simulink model "TestStructure"  (R2023b)
settings: Solver=FixedStepDiscrete  StartTime=0.0  StopTime=inf  FixedStep=SampleTime  RelTol=1e-3
InitFcn:
  | SampleTime = 0.001;
  | ButtonValue=0;
  | load("BusConfig.mat");
undefined symbols (not defined in the file): DiscIntNeverNeededParam
libraries: slrealtimeethercatlib x219, dspfdesign x28, dspstat3 x23, simulink x21, slpidlib x10, dspswit3 x8, commfilt2 x2, dspsigops x1
(part 1 of 8)
settings Model: SimulationMode=external  ExtModeEnableFloating=off  Creator=My-Dell-PC  LastModifiedBy=My-Dell-PC
settings SolverCC: ConcurrentTasks=on  PositivePriorityOrder=on
settings OptimizationCC: BlockReduction=off  OptimizeBlockIOStorage=off  ReuseModelBlockBuffer=off
settings DebuggingCC: TasksWithSamePriorityMsg=none
settings HardwareCC: ProdBitPerLong=64  ProdLongLongMode=on  ProdHWDeviceType=Intel->x86-64 (Linux 64)
settings RTWCC: Description=Simulink Real-Time  SystemTargetFile=slrealtime.tlc  TemplateMakefile=slrealtime_default_tmf  Toolchain=Simulink Real-Time Toolchain  BuildConfiguration=Faster Runs  CodeExecutionProfiling=on  TargetLang=C++
settings CodeAppCC: MaxIdLength=128

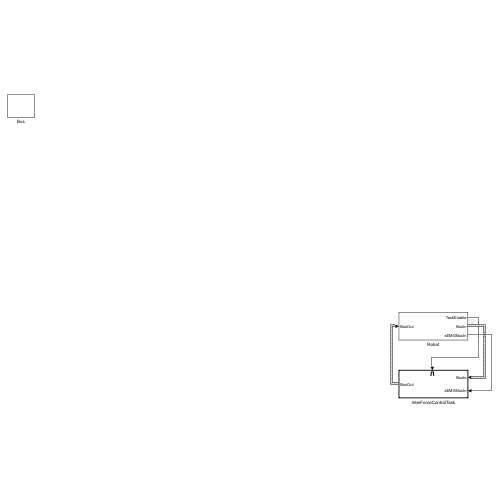
[thumbnail: Simulink's stored preview of the top-level diagram]
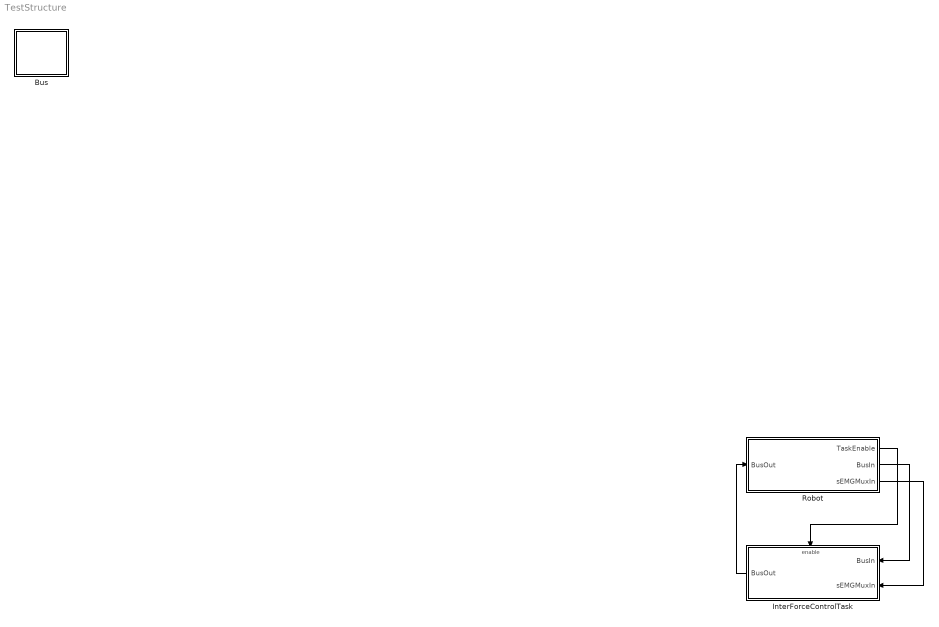
== system TestStructure ==
  Bus : Subsystem  mask{Parameter1=0}
  InterForceControlTask : Subsystem  TreatAsAtomicUnit=on
  Robot : Subsystem  InitFcn=|
      | LeftHipMotorPosDefault = -134217728;                %Unit: Cnt
      | RightHipMotorPosDefault = -134217728;               %Unit: Cnt
      | LeftHipMotor_InitPos_Degree = 185;           %Unit: Degree
      | RightHipMotor_InitPos_Degree = 58;          %Unit: Degree
      | LeftHipMotorSensorCh1FDirection = -1;       %Unit: None        1 or -1, 0 for not use
      | RightHipMotorSensorCh1FDirection = 1;      %Unit: None        1 or -1, 0 for not use
      | LeftHipMotorPosProtectUpperLim = 0;        %Unit: Degree      both Upper and lower lim config to 0 for no protect
      | LeftHipMotorPosProtectLowerLim = 0;        %Unit: Degree      both Upper and lower lim config to 0 for no protect
      | RightHipMotorPosProtectUpperLim = 0;       %Unit: Degree      both Upper and lower lim config to 0 for no protect
      | RightHipMotorPosProtectLowerLim = 0;       %Unit: Degree      both Upper and lower lim config to 0 for no protect
  wires:
  Robot/2(BusIn) -> InterForceControlTask/1(BusIn)
  Robot/1(TaskEnable) -> InterForceControlTask/Enable
  InterForceControlTask/1(BusOut) -> Robot/1(BusOut)
  Robot/3(sEMGMuxIn) -> InterForceControlTask/2(sEMGMuxIn)

== system TestStructure/Bus ==
  Subsystem : Subsystem
  Subsystem1 : Subsystem
  Subsystem4 : Subsystem
  Subsystem5 : Subsystem
  Subsystem6 : Subsystem
  Subsystem7 : Subsystem

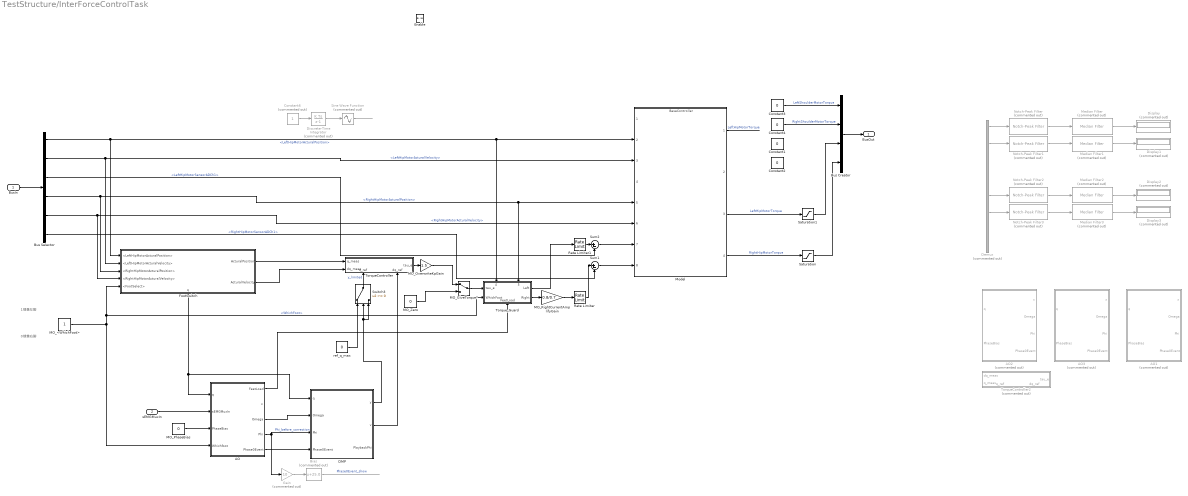
== system TestStructure/InterForceControlTask ==
  note: 0镜像右脚
  note: 1镜像左脚
  BusIn : Inport  OutDataTypeStr=Bus: SensingBusNew  BusOutputAsStruct=on
  sEMGMuxIn : Inport  Port=2
  Enable : EnablePort
  AO : Subsystem
  AO1 : Subsystem  Commented=on
  AO2 : Subsystem  Commented=on
  AO3 : Subsystem  Commented=on
  Bias : Bias  Commented=on  Bias=25.0  SaturateOnIntegerOverflow=off
  Bus Creator : BusCreator  Inputs=4  OutDataTypeStr=Bus: ControlBusNew  NonVirtualBus=on
  Bus Selector : BusSelector  OutputSignals=LeftHipMotorActuralPosition,LeftHipMotorActuralVelocity,LeftHipMotorSensorADCh1,RightHipMotorActuralPosition,RightHipMotorActuralVelocity,RightHipMotorSensorADCh1
  Constant{1..4} (4 alike) : Constant  Value=0
  Constant6 : Constant  Commented=on
  DMP : Subsystem
  Demux : Demux  Commented=on  Outputs=8
  Discrete-Time Integrator : DiscreteIntegrator  Commented=on  SampleTime=-1  ICPrevOutput=DiscIntNeverNeededParam  ICPrevScaledInput=DiscIntNeverNeededParam
  Display{,1..3} (4 alike) : Display  Commented=on
  FootSwitch : Subsystem
      settings: PortSchema="{\"entries\":[{\"content\":{\"sides\":[{\"content\":{\"connectorIds\":[\"In1\",\"In2\",\"In3\",\"In4\",\"In5\"]},\"type\":\"ConnectorPlacement.EquallySpacedRectSide\",\"uuid\":\"7ecdb0d1-44f7-4cb8-804e-f6057fee00e3\"},{\"content\":{\"connectorIds\":[\"Out1\",\"Out2\"],\"side\":\"RIGHT\"},\"type\":\"ConnectorPlacement.EquallySpacedRectSide\",\"uuid\":\"b63e60e1-496e-4124-94d3-4dbeb666215a\"},{\"content\":{\"side\":\"TOP\"},\"type\":\"ConnectorPlacement.EquallySpacedRectSide\",\"uuid\":\"11a332ee-5b07-4fe6-93fe-1398bc56bf27\"},{\"content\":{\"connectorIds\":[\"Out3\"],\"side\":\"BOTTOM\"},\"type\":\"ConnectorPlacement.EquallySpacedRectSide\",\"uuid\":\"ff7a2680-cae9-4957-8a73-46cd45583629\"}]},\"type\":\"ConnectorPlacement.EquallySpacedConnector\",\"uuid\":\"1c496143-d045-4bb8-a283-2b92538bf384\"}],\"packageUris\":[\"http://schema.mathworks.com/mf0/Connector/R2020b\"],\"version\":\"1.0\"}"
  Gain : Gain  Commented=on  Gain=10
  MO_<WhichFoot> : Constant
  MO_GiveTorque? : ManualSwitch
  MO_OverwriteKpGain : Gain  Gain=1.5
  MO_PhaseBias : Constant  Value=0
  MO_RightCurrentAmplifyGain : Gain  Gain=0.8/0.7
  MO_Zero : Constant  Value=0
  Median Filter{,1..3} (4 alike) : dspstat3/Median Filter  Commented=on  WindowLength=5  SimulateUsing=Interpreted execution
      settings: LibrarySourceBlock=|
      | dspfdesign/Median
      | Filter
  Model : ModelReference  ModelNameDialog=BaseController.slxp  ModelReferenceVersion=3.421  CopyOfModelProtected=on
  Notch-Peak Filter{,1..3} (4 alike) : dspfdesign/Notch-Peak Filter  Commented=on  Specification=Quality factor and center frequency  BandwidthPort=on  Bandwidth=2205  QualityFactorPort=off  QualityFactor=5  CenterFrequencyPort=off  CenterFrequency=50  BandwidthCoefficientPort=off  BandwidthCoefficient=0.72654  CenterFrequencyCoefficientPort=off  CenterFrequencyCoefficient=0  Output=Notch  InheritSampleRate=off  SampleRate=1000  SimulateUsing=Code generation
  Rate Limiter : RateLimiter  RisingSlewLimit=60  FallingSlewLimit=-60  SampleTimeMode=inherited
  Rate Limiter1 : RateLimiter  RisingSlewLimit=60  FallingSlewLimit=-60  SampleTimeMode=inherited
  Saturation : Saturate  UpperLimit=20  LowerLimit=-20
  Saturation1 : Saturate  UpperLimit=20  LowerLimit=-20
  Sine Wave Function : Sin  Commented=on  TimeSource=Use external signal  Amplitude=30  Bias=-30  Frequency=2*pi*0.5  Phase=0.5*pi  SampleTime=0
  Sum1 : Sum  Inputs=|+-
  Sum2 : Sum  Inputs=|+-
  Switch3 : Switch  SaturateOnIntegerOverflow=off  InputSameDT=off
  TorqueController : Subsystem
      settings: PortSchema="{\"entries\":[{\"content\":{\"sides\":[{\"content\":{\"connectorIds\":[\"In1\",\"In2\"]},\"type\":\"ConnectorPlacement.EquallySpacedRectSide\",\"uuid\":\"a70f4d3f-71f0-4d44-86b2-84ae6c965d36\"},{\"content\":{\"connectorIds\":[\"Out1\"],\"side\":\"RIGHT\"},\"type\":\"ConnectorPlacement.EquallySpacedRectSide\",\"uuid\":\"94df1563-b6d2-45fb-b198-7d0905a4894a\"},{\"content\":{\"side\":\"TOP\"},\"type\":\"ConnectorPlacement.EquallySpacedRectSide\",\"uuid\":\"a4abfadc-4e4d-4360-b10c-eb4f639dc4a4\"},{\"content\":{\"connectorIds\":[\"In3\",\"In4\"],\"side\":\"BOTTOM\"},\"type\":\"ConnectorPlacement.EquallySpacedRectSide\",\"uuid\":\"0f098f5c-7d68-4c78-935c-71623c896b5b\"}]},\"type\":\"ConnectorPlacement.EquallySpacedConnector\",\"uuid\":\"e58753f5-b0b7-4189-98c1-665b5fbcbb59\"}],\"packageUris\":[\"http://schema.mathworks.com/mf0/Connector/R2020b\"],\"version\":\"1.0\"}"
  TorqueController2 : Subsystem  Commented=on
      settings: PortSchema="{\"entries\":[{\"content\":{\"sides\":[{\"content\":{\"connectorIds\":[\"In1\",\"In2\"]},\"type\":\"ConnectorPlacement.EquallySpacedRectSide\",\"uuid\":\"a70f4d3f-71f0-4d44-86b2-84ae6c965d36\"},{\"content\":{\"connectorIds\":[\"Out1\"],\"side\":\"RIGHT\"},\"type\":\"ConnectorPlacement.EquallySpacedRectSide\",\"uuid\":\"94df1563-b6d2-45fb-b198-7d0905a4894a\"},{\"content\":{\"side\":\"TOP\"},\"type\":\"ConnectorPlacement.EquallySpacedRectSide\",\"uuid\":\"a4abfadc-4e4d-4360-b10c-eb4f639dc4a4\"},{\"content\":{\"connectorIds\":[\"In3\",\"In4\"],\"side\":\"BOTTOM\"},\"type\":\"ConnectorPlacement.EquallySpacedRectSide\",\"uuid\":\"0f098f5c-7d68-4c78-935c-71623c896b5b\"}]},\"type\":\"ConnectorPlacement.EquallySpacedConnector\",\"uuid\":\"e58753f5-b0b7-4189-98c1-665b5fbcbb59\"}],\"packageUris\":[\"http://schema.mathworks.com/mf0/Connector/R2020b\"],\"version\":\"1.0\"}"
  Torque_Guard : Subsystem
      settings: PortSchema="{\"entries\":[{\"content\":{\"sides\":[{\"content\":{\"connectorIds\":[\"In1\"]},\"type\":\"ConnectorPlacement.EquallySpacedRectSide\",\"uuid\":\"1d23c2d1-211b-4c47-b88b-c8f5a33413bd\"},{\"content\":{\"connectorIds\":[\"In4\",\"In5\"],\"side\":\"RIGHT\"},\"type\":\"ConnectorPlacement.EquallySpacedRectSide\",\"uuid\":\"4048f38c-2874-4094-b8f6-a75ec179b5c6\"},{\"content\":{\"connectorIds\":[\"In2\",\"In3\"],\"side\":\"TOP\"},\"type\":\"ConnectorPlacement.EquallySpacedRectSide\",\"uuid\":\"5dc62aa6-b4b6-4778-a65d-61d1e67b5e0a\"},{\"content\":{\"connectorIds\":[\"Out1\",\"Out2\"],\"side\":\"BOTTOM\"},\"type\":\"ConnectorPlacement.EquallySpacedRectSide\",\"uuid\":\"4577c0a2-eb02-4748-b343-e51a2d06d9c8\"}]},\"type\":\"ConnectorPlacement.EquallySpacedConnector\",\"uuid\":\"b262622a-1d3e-4ad6-baa7-9b3b8428161e\"}],\"packageUris\":[\"http://schema.mathworks.com/mf0/Connector/R2020b\"],\"version\":\"1.0\"}"
  ref_q_max : Constant  Value=0
  BusOut : Outport  OutDataTypeStr=Bus: ControlBusNew  BusOutputAsStruct=on
  wires:
  Bus Creator/1 -> BusOut/1
  Model/1 -> ?  "LeftHipMotorTorque"
  BusIn/1 -> Bus Selector/1
  Constant3/1 -> Bus Creator/1  "LeftShoulderMotorTorque"
  Model/4 -> Saturation/1  "RightHipMotorTorque"
  Constant4/1 -> Bus Creator/2  "RightShoulderMotorTorque"
  Sum2/1 -> Model/7
  Bus Selector/4 -> FootSwitch/3(<RightHipMotorActuralPosition>), Torque_Guard/5(<RightHipMotorActuralPosition>), Model/5  "<RightHipMotorActuralPosition>"
  Bus Selector/5 -> FootSwitch/4(<RightHipMotorActuralVelocity>), Model/6  "<RightHipMotorActuralVelocity>"
  Bus Selector/2 -> FootSwitch/2(<LeftHipMotorActuralVelocity>), Model/3  "<LeftHipMotorActuralVelocity>"
  Bus Selector/3 -> Sum2/2  "<LeftHipMotorSensorADCh1>"
  Bus Selector/6 -> Sum1/2  "<RightHipMotorSensorADCh1>"
  Constant6/1 -> Discrete-Time Integrator/1
  Discrete-Time Integrator/1 -> Sine Wave Function/1
  Sine Wave Function/1 -> ?
  Median Filter3/1 -> Display3/1
  Notch-Peak Filter2/1 -> Median Filter2/1
  Demux/2 -> Notch-Peak Filter1/1
  Median Filter1/1 -> Display1/1
  Notch-Peak Filter3/1 -> Median Filter3/1
  Notch-Peak Filter/1 -> Median Filter/1
  Demux/5 -> Notch-Peak Filter2/1
  Median Filter2/1 -> Display2/1
  Demux/1 -> Notch-Peak Filter/1
  Median Filter/1 -> Display/1
  Notch-Peak Filter1/1 -> Median Filter1/1
  Demux/6 -> Notch-Peak Filter3/1
  MO_PhaseBias/1 -> AO/3(PhaseBias)
  AO/4(Phi) -> DMP/3(Phi), Gain/1  "Phi_before_correction"
  AO/5(Phase0Event) -> DMP/4(Phase0Event)
  DMP/2(v) -> TorqueController/4(dq_ref)
  AO/3(Omega) -> DMP/2(Omega)
  Bus Selector/1 -> FootSwitch/1(<LeftHipMotorActuralPosition>), Model/2, Torque_Guard/4(<LeftHipMotorActuralPosition>)  "<LeftHipMotorActuralPosition>"
  Saturation/1 -> Bus Creator/4
  Model/3 -> Saturation1/1  "LeftHipMotorTorque"
  Saturation1/1 -> Bus Creator/3
  Gain/1 -> Bias/1
  Bias/1 -> ?  "Phase0Event_show"
  MO_Zero/1 -> MO_GiveTorque?/2
  TorqueController/1(tau_e) -> MO_OverwriteKpGain/1
  Sum1/1 -> Model/8
  sEMGMuxIn/1 -> AO/2(sEMGMuxIn)
  FootSwitch/3(q) -> DMP/1(q), AO/1(q)
  FootSwitch/1(ActuralPosition) -> TorqueController/1(q_meas)
  FootSwitch/2(ActuralVelocity) -> TorqueController/2(dq_meas)
  MO_GiveTorque?/1 -> Torque_Guard/3(tau_e)
  Torque_Guard/2(Left) -> Rate Limiter1/1
  Torque_Guard/1(Right) -> MO_RightCurrentAmplifyGain/1
  MO_<WhichFoot>/1 -> FootSwitch/5(<FootSelect>), Torque_Guard/2(WhichFoot), AO/4(Whichfoot)  "<WhichFoot>"
  Rate Limiter/1 -> Sum1/1
  AO/1(FeetLoad) -> Torque_Guard/1(FeetLoad)
  DMP/1(y) -> Switch3/3, Switch3/2
  ref_q_max/1 -> Switch3/1
  Switch3/1 -> TorqueController/3(q_ref)  "y_limited"
  MO_OverwriteKpGain/1 -> MO_GiveTorque?/1
  MO_RightCurrentAmplifyGain/1 -> Rate Limiter/1
  Rate Limiter1/1 -> Sum2/1

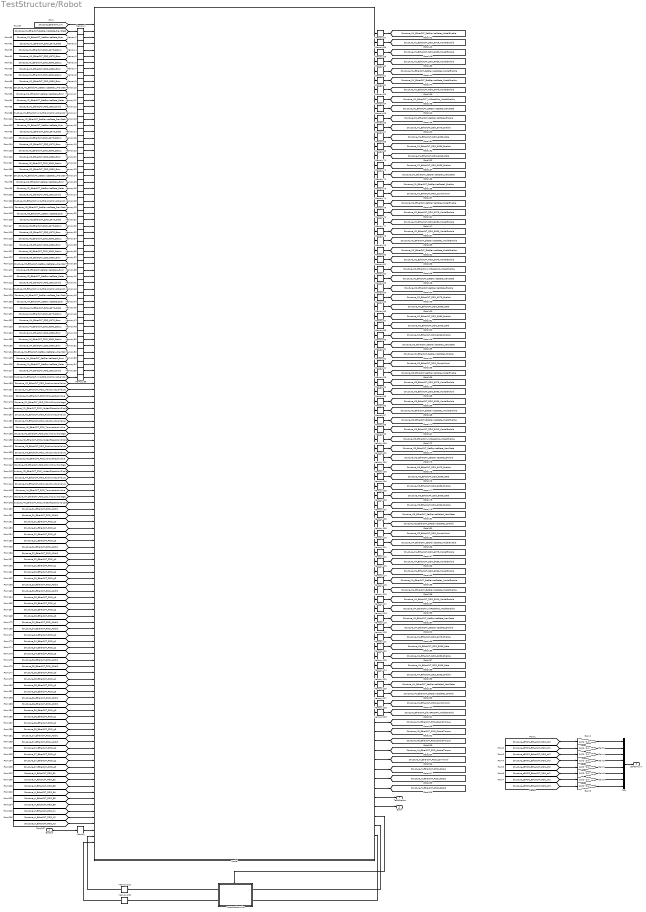
== system TestStructure/Robot ==
  BusOut : Inport
  Gain{1,3..9} (8 alike) : Gain  Gain=10/(2^24)
  Memory{,1..131} (132 alike) : Memory
  Model : ModelReference  ModelNameDialog=Robot2.slxp  ModelReferenceVersion=3.62  CopyOfModelProtected=on
  MotorPositonInit1 : Subsystem
  Mux : Mux  Inputs=8
  TaskEnable : Outport
  BusIn : Outport  Port=2
  sEMGMuxIn : Outport  Port=3
  tag scope: Structure_EtherCAT_SlavePDORW_ModelEnable=global, Structure_H_EtherCAT_PDO_Command=global, Structure_H_EtherCAT_PDO_Data1=global, Structure_H_EtherCAT_PDO_Data2=global, Structure_H_EtherCAT_PDO_Data3=global, Structure_M1_EtherCAT_GetDeviceState_ModelEnable=global, Structure_M1_EtherCAT_InitReadPos_ModelEnable=global, Structure_M1_EtherCAT_PDO_6040_ModelEnable=global, Structure_M1_EtherCAT_PDO_ControlWord=global, Structure_M1_EtherCAT_PDO_DesireTorque=global, Structure_M1_EtherCAT_SDO_6060_Data=global, Structure_M1_EtherCAT_SDO_6060_Enable=global, Structure_M1_EtherCAT_SDO_6060_ModelEnable=global, Structure_M1_EtherCAT_SDO_6075_Enable=global, Structure_M1_EtherCAT_SDO_6075_ModelEnable=global, Structure_M1_EtherCAT_SDO_6080_Data=global, Structure_M1_EtherCAT_SDO_6080_Enable=global, Structure_M1_EtherCAT_SDO_6080_ModelEnable=global, Structure_M1_EtherCAT_SetDeviceState1_Enable=global, Structure_M1_EtherCAT_SetDeviceState1_ModelEnable=global, Structure_M1_EtherCAT_SetDeviceState1_NewState=global, Structure_M1_EtherCAT_SetDeviceState_Enable=global, Structure_M1_EtherCAT_SetDeviceState_ModelEnable=global, Structure_M1_EtherCAT_SetDeviceState_NewState=global, Structure_M2_EtherCAT_GetDeviceState_ModelEnable=global, Structure_M2_EtherCAT_InitReadPos_ModelEnable=global, Structure_M2_EtherCAT_PDO_6040_ModelEnable=global, Structure_M2_EtherCAT_PDO_ControlWord=global, Structure_M2_EtherCAT_PDO_DesireTorque=global, Structure_M2_EtherCAT_SDO_6060_Data=global, Structure_M2_EtherCAT_SDO_6060_Enable=global, Structure_M2_EtherCAT_SDO_6060_ModelEnable=global, Structure_M2_EtherCAT_SDO_6075_Enable=global, Structure_M2_EtherCAT_SDO_6075_ModelEnable=global, Structure_M2_EtherCAT_SDO_6080_Data=global, Structure_M2_EtherCAT_SDO_6080_Enable=global, Structure_M2_EtherCAT_SDO_6080_ModelEnable=global, Structure_M2_EtherCAT_SetDeviceState1_Enable=global, Structure_M2_EtherCAT_SetDeviceState1_ModelEnable=global, Structure_M2_EtherCAT_SetDeviceState1_NewState=global, Structure_M2_EtherCAT_SetDeviceState_Enable=global, Structure_M2_EtherCAT_SetDeviceState_ModelEnable=global, Structure_M2_EtherCAT_SetDeviceState_NewState=global, Structure_M3_EtherCAT_GetDeviceState_ModelEnable=global, Structure_M3_EtherCAT_InitReadPos_ModelEnable=global, Structure_M3_EtherCAT_PDO_6040_ModelEnable=global, Structure_M3_EtherCAT_PDO_ControlWord=global, Structure_M3_EtherCAT_PDO_DesireTorque=global, Structure_M3_EtherCAT_SDO_6060_Data=global, Structure_M3_EtherCAT_SDO_6060_Enable=global, Structure_M3_EtherCAT_SDO_6060_ModelEnable=global, Structure_M3_EtherCAT_SDO_6075_Enable=global, Structure_M3_EtherCAT_SDO_6075_ModelEnable=global, Structure_M3_EtherCAT_SDO_6080_Data=global, Structure_M3_EtherCAT_SDO_6080_Enable=global, Structure_M3_EtherCAT_SDO_6080_ModelEnable=global, Structure_M3_EtherCAT_SetDeviceState1_Enable=global, Structure_M3_EtherCAT_SetDeviceState1_ModelEnable=global, Structure_M3_EtherCAT_SetDeviceState1_NewState=global, Structure_M3_EtherCAT_SetDeviceState_Enable=global, Structure_M3_EtherCAT_SetDeviceState_ModelEnable=global, Structure_M3_EtherCAT_SetDeviceState_NewState=global, Structure_M4_EtherCAT_GetDeviceState_ModelEnable=global, Structure_M4_EtherCAT_InitReadPos_ModelEnable=global, Structure_M4_EtherCAT_PDO_6040_ModelEnable=global, Structure_M4_EtherCAT_PDO_ControlWord=global, Structure_M4_EtherCAT_PDO_DesireTorque=global, Structure_M4_EtherCAT_SDO_6060_Data=global, Structure_M4_EtherCAT_SDO_6060_Enable=global, Structure_M4_EtherCAT_SDO_6060_ModelEnable=global, Structure_M4_EtherCAT_SDO_6075_Enable=global, Structure_M4_EtherCAT_SDO_6075_ModelEnable=global, Structure_M4_EtherCAT_SDO_6080_Data=global, Structure_M4_EtherCAT_SDO_6080_Enable=global, Structure_M4_EtherCAT_SDO_6080_ModelEnable=global, Structure_M4_EtherCAT_SetDeviceState1_Enable=global, Structure_M4_EtherCAT_SetDeviceState1_ModelEnable=global, Structure_M4_EtherCAT_SetDeviceState1_NewState=global, Structure_M4_EtherCAT_SetDeviceState_Enable=global, Structure_M4_EtherCAT_SetDeviceState_ModelEnable=global, Structure_M4_EtherCAT_SetDeviceState_NewState=global
  wires:
  [Structure_EtherCAT_Init] -> Model/1
  [Structure_M1_EtherCAT_SetDeviceState_PrevState] -> Memory1/1
  [Structure_M1_EtherCAT_SetDeviceState_Error] -> Memory2/1
  [Structure_M1_EtherCAT_SDO_6075_Data] -> Memory3/1
  Model/1 -> Memory57/1
  Model/2 -> Memory58/1
  Model/3 -> Memory59/1
  Model/4 -> Memory60/1
  Model/5 -> Memory61/1
  Model/6 -> Memory62/1
  [Structure_M1_EtherCAT_SDO_6075_Status] -> Memory4/1
  [Structure_M1_EtherCAT_SDO_6075_Error] -> Memory5/1
  [Structure_M1_EtherCAT_SDO_6080_Status] -> Memory6/1
  [Structure_M1_EtherCAT_SDO_6080_Error] -> Memory7/1
  [Structure_M1_EtherCAT_SDO_6060_Status] -> Memory8/1
  [Structure_M1_EtherCAT_SDO_6060_Error] -> Memory9/1
  [Structure_M1_EtherCAT_SetDeviceState1_PrevState] -> Memory10/1
  [Structure_M1_EtherCAT_SetDeviceState1_Error] -> Memory11/1
  [Structure_M1_EtherCAT_GetDeviceState_State] -> Memory12/1
  [Structure_M1_EtherCAT_PDO_StatusWord] -> Memory13/1
  [Structure_M1_EtherCAT_Init_PDO_PositionActualValue] -> Memory14/1
  [Structure_M2_EtherCAT_SetDeviceState_PrevState] -> Memory15/1
  [Structure_M2_EtherCAT_SetDeviceState_Error] -> Memory16/1
  [Structure_M2_EtherCAT_SDO_6075_Data] -> Memory17/1
  [Structure_M2_EtherCAT_SDO_6075_Status] -> Memory18/1
  [Structure_M2_EtherCAT_SDO_6075_Error] -> Memory19/1
  [Structure_M2_EtherCAT_SDO_6080_Status] -> Memory20/1
  [Structure_M2_EtherCAT_SDO_6080_Error] -> Memory21/1
  [Structure_M2_EtherCAT_SDO_6060_Status] -> Memory22/1
  [Structure_M2_EtherCAT_SDO_6060_Error] -> Memory23/1
  [Structure_M2_EtherCAT_SetDeviceState1_PrevState] -> Memory24/1
  [Structure_M2_EtherCAT_SetDeviceState1_Error] -> Memory25/1
  [Structure_M2_EtherCAT_GetDeviceState_State] -> Memory26/1
  [Structure_M2_EtherCAT_PDO_StatusWord] -> Memory27/1
  [Structure_M2_EtherCAT_Init_PDO_PositionActualValue] -> Memory28/1
  [Structure_M3_EtherCAT_SetDeviceState_PrevState] -> Memory29/1
  [Structure_M3_EtherCAT_SetDeviceState_Error] -> Memory30/1
  [Structure_M3_EtherCAT_SDO_6075_Data] -> Memory31/1
  [Structure_M3_EtherCAT_SDO_6075_Status] -> Memory32/1
  [Structure_M3_EtherCAT_SDO_6075_Error] -> Memory33/1
  [Structure_M3_EtherCAT_SDO_6080_Status] -> Memory34/1
  [Structure_M3_EtherCAT_SDO_6080_Error] -> Memory35/1
  [Structure_M3_EtherCAT_SDO_6060_Status] -> Memory36/1
  [Structure_M3_EtherCAT_SDO_6060_Error] -> Memory37/1
  [Structure_M3_EtherCAT_SetDeviceState1_PrevState] -> Memory38/1
  [Structure_M3_EtherCAT_SetDeviceState1_Error] -> Memory39/1
  [Structure_M3_EtherCAT_GetDeviceState_State] -> Memory40/1
  [Structure_M3_EtherCAT_PDO_StatusWord] -> Memory41/1
  [Structure_M3_EtherCAT_Init_PDO_PositionActualValue] -> Memory42/1
  [Structure_M4_EtherCAT_SetDeviceState_PrevState] -> Memory43/1
  [Structure_M4_EtherCAT_SetDeviceState_Error] -> Memory44/1
  [Structure_M4_EtherCAT_SDO_6075_Data] -> Memory45/1
  [Structure_M4_EtherCAT_SDO_6075_Status] -> Memory46/1
  [Structure_M4_EtherCAT_SDO_6075_Error] -> Memory47/1
  [Structure_M4_EtherCAT_SDO_6080_Status] -> Memory48/1
  [Structure_M4_EtherCAT_SDO_6080_Error] -> Memory49/1
  [Structure_M4_EtherCAT_SDO_6060_Status] -> Memory50/1
  [Structure_M4_EtherCAT_SDO_6060_Error] -> Memory51/1
  [Structure_M4_EtherCAT_SetDeviceState1_PrevState] -> Memory52/1
  [Structure_M4_EtherCAT_SetDeviceState1_Error] -> Memory53/1
  [Structure_M4_EtherCAT_GetDeviceState_State] -> Memory54/1
  [Structure_M4_EtherCAT_PDO_StatusWord] -> Memory55/1
  [Structure_M4_EtherCAT_Init_PDO_PositionActualValue] -> Memory56/1
  Model/73 -> Memory129/1
  Model/72 -> Memory128/1
  Model/71 -> Memory127/1
  Model/70 -> Memory126/1
  Model/69 -> Memory125/1
  Model/68 -> Memory124/1
  Model/67 -> Memory123/1
  Model/66 -> Memory122/1
  Model/65 -> Memory121/1
  Model/64 -> Memory120/1
  Model/63 -> Memory119/1
  Model/62 -> Memory118/1
  Model/61 -> Memory117/1
  Model/60 -> Memory116/1
  Model/59 -> Memory115/1
  Model/58 -> Memory114/1
  Model/57 -> Memory113/1
  Model/56 -> Memory112/1
  Model/55 -> Memory111/1
  Model/54 -> Memory110/1
  Model/53 -> Memory109/1
  Model/52 -> Memory108/1
  Model/51 -> Memory107/1
  Model/50 -> Memory106/1
  Model/49 -> Memory105/1
  Model/48 -> Memory104/1
  Model/47 -> Memory103/1
  Model/46 -> Memory102/1
  Model/45 -> Memory101/1
  Model/44 -> Memory100/1
  Model/43 -> Memory99/1
  Model/42 -> Memory98/1
  Model/41 -> Memory97/1
  Model/40 -> Memory96/1
  Model/39 -> Memory95/1
  Model/38 -> Memory94/1
  Model/37 -> Memory93/1
  Model/36 -> Memory92/1
  Model/35 -> Memory91/1
  Model/34 -> Memory90/1
  Model/33 -> Memory89/1
  Model/32 -> Memory88/1
  Model/31 -> Memory87/1
  Model/30 -> Memory86/1
  Model/29 -> Memory85/1
  Model/28 -> Memory84/1
  Model/27 -> Memory83/1
  Model/26 -> Memory82/1
  Model/25 -> Memory81/1
  Model/24 -> Memory80/1
  Model/23 -> Memory79/1
  Model/22 -> Memory78/1
  Model/21 -> Memory77/1
  Model/20 -> Memory76/1
  Model/19 -> Memory75/1
  Model/18 -> Memory74/1
  Model/17 -> Memory73/1
  Model/16 -> Memory72/1
  Model/15 -> Memory71/1
  Model/14 -> Memory70/1
  Model/13 -> Memory69/1
  Model/12 -> Memory68/1
  Model/11 -> Memory67/1
  Model/10 -> Memory66/1
  Model/9 -> Memory65/1
  Model/8 -> Memory64/1
  Model/7 -> Memory63/1
  Memory1/1 -> Model/2
  Memory2/1 -> Model/3
  Memory3/1 -> Model/4
  Memory4/1 -> Model/5
  Memory5/1 -> Model/6
  Memory6/1 -> Model/7
  Memory7/1 -> Model/8
  Memory8/1 -> Model/9
  Memory9/1 -> Model/10
  Memory10/1 -> Model/11
  Memory11/1 -> Model/12
  Memory12/1 -> Model/13
  Memory13/1 -> Model/14
  Memory14/1 -> Model/15
  Memory15/1 -> Model/16
  Memory16/1 -> Model/17
  Memory17/1 -> Model/18
  Memory18/1 -> Model/19
  Memory19/1 -> Model/20
  Memory20/1 -> Model/21
  Memory21/1 -> Model/22
  Memory22/1 -> Model/23
  Memory23/1 -> Model/24
  Memory24/1 -> Model/25
  Memory25/1 -> Model/26
  Memory26/1 -> Model/27
  Memory27/1 -> Model/28
  Memory28/1 -> Model/29
  Memory29/1 -> Model/30
  Memory30/1 -> Model/31
  Memory31/1 -> Model/32
  Memory32/1 -> Model/33
  Memory33/1 -> Model/34
  Memory34/1 -> Model/35
  Memory35/1 -> Model/36
  Memory36/1 -> Model/37
  Memory37/1 -> Model/38
  Memory38/1 -> Model/39
  Memory39/1 -> Model/40
  Memory40/1 -> Model/41
  Memory41/1 -> Model/42
  Memory42/1 -> Model/43
  Memory43/1 -> Model/44
  Memory44/1 -> Model/45
  Memory45/1 -> Model/46
  Memory46/1 -> Model/47
  Memory47/1 -> Model/48
  Memory48/1 -> Model/49
  Memory49/1 -> Model/50
  Memory50/1 -> Model/51
  Memory51/1 -> Model/52
  Memory52/1 -> Model/53
  Memory53/1 -> Model/54
  Memory54/1 -> Model/55
  Memory55/1 -> Model/56
  Memory56/1 -> Model/57
  Memory57/1 -> [Structure_M1_EtherCAT_SetDeviceState_ModelEnable]
  Memory58/1 -> [Structure_M1_EtherCAT_SDO_6075_ModelEnable]
  Memory59/1 -> [Structure_M1_EtherCAT_SDO_6080_ModelEnable]
  Memory60/1 -> [Structure_M1_EtherCAT_SDO_6060_ModelEnable]
  Memory61/1 -> [Structure_M1_EtherCAT_SetDeviceState1_ModelEnable]
  Memory62/1 -> [Structure_M1_EtherCAT_GetDeviceState_ModelEnable]
  Memory63/1 -> [Structure_M1_EtherCAT_PDO_6040_ModelEnable]
  Memory64/1 -> [Structure_M1_EtherCAT_InitReadPos_ModelEnable]
  Memory65/1 -> [Structure_M1_EtherCAT_SetDeviceState_NewState]
  Memory66/1 -> [Structure_M1_EtherCAT_SetDeviceState_Enable]
  Memory67/1 -> [Structure_M1_EtherCAT_SDO_6075_Enable]
  Memory68/1 -> [Structure_M1_EtherCAT_SDO_6080_Data]
  Memory69/1 -> [Structure_M1_EtherCAT_SDO_6080_Enable]
  Memory73/1 -> [Structure_M1_EtherCAT_SetDeviceState1_Enable]
  Memory71/1 -> [Structure_M1_EtherCAT_SDO_6060_Enable]
  Memory74/1 -> [Structure_M1_EtherCAT_PDO_ControlWord]
  Memory70/1 -> [Structure_M1_EtherCAT_SDO_6060_Data]
  Memory72/1 -> [Structure_M1_EtherCAT_SetDeviceState1_NewState]
  Memory76/1 -> [Structure_M2_EtherCAT_SDO_6075_ModelEnable]
  Memory78/1 -> [Structure_M2_EtherCAT_SDO_6060_ModelEnable]
  Memory79/1 -> [Structure_M2_EtherCAT_SetDeviceState1_ModelEnable]
  Memory77/1 -> [Structure_M2_EtherCAT_SDO_6080_ModelEnable]
  Memory75/1 -> [Structure_M2_EtherCAT_SetDeviceState_ModelEnable]
  Memory80/1 -> [Structure_M2_EtherCAT_GetDeviceState_ModelEnable]
  Memory81/1 -> [Structure_M2_EtherCAT_PDO_6040_ModelEnable]
  Memory82/1 -> [Structure_M2_EtherCAT_InitReadPos_ModelEnable]
  Memory83/1 -> [Structure_M2_EtherCAT_SetDeviceState_NewState]
  Memory84/1 -> [Structure_M2_EtherCAT_SetDeviceState_Enable]
  Memory85/1 -> [Structure_M2_EtherCAT_SDO_6075_Enable]
  Memory88/1 -> [Structure_M2_EtherCAT_SDO_6060_Data]
  Memory86/1 -> [Structure_M2_EtherCAT_SDO_6080_Data]
  Memory87/1 -> [Structure_M2_EtherCAT_SDO_6080_Enable]
  Memory89/1 -> [Structure_M2_EtherCAT_SDO_6060_Enable]
  Memory90/1 -> [Structure_M2_EtherCAT_SetDeviceState1_NewState]
  Memory91/1 -> [Structure_M2_EtherCAT_SetDeviceState1_Enable]
  Memory92/1 -> [Structure_M2_EtherCAT_PDO_ControlWord]
  Memory93/1 -> [Structure_M3_EtherCAT_SetDeviceState_ModelEnable]
  Memory94/1 -> [Structure_M3_EtherCAT_SDO_6075_ModelEnable]
  Memory98/1 -> [Structure_M3_EtherCAT_GetDeviceState_ModelEnable]
  Memory99/1 -> [Structure_M3_EtherCAT_PDO_6040_ModelEnable]
  Memory97/1 -> [Structure_M3_EtherCAT_SetDeviceState1_ModelEnable]
  Memory96/1 -> [Structure_M3_EtherCAT_SDO_6060_ModelEnable]
  Memory95/1 -> [Structure_M3_EtherCAT_SDO_6080_ModelEnable]
  Memory103/1 -> [Structure_M3_EtherCAT_SDO_6075_Enable]
  Memory104/1 -> [Structure_M3_EtherCAT_SDO_6080_Data]
  Memory102/1 -> [Structure_M3_EtherCAT_SetDeviceState_Enable]
  Memory101/1 -> [Structure_M3_EtherCAT_SetDeviceState_NewState]
  Memory100/1 -> [Structure_M3_EtherCAT_InitReadPos_ModelEnable]
  Memory106/1 -> [Structure_M3_EtherCAT_SDO_6060_Data]
  Memory105/1 -> [Structure_M3_EtherCAT_SDO_6080_Enable]
  Memory109/1 -> [Structure_M3_EtherCAT_SetDeviceState1_Enable]
  Memory108/1 -> [Structure_M3_EtherCAT_SetDeviceState1_NewState]
  Memory107/1 -> [Structure_M3_EtherCAT_SDO_6060_Enable]
  Memory113/1 -> [Structure_M4_EtherCAT_SDO_6080_ModelEnable]
  Memory111/1 -> [Structure_M4_EtherCAT_SetDeviceState_ModelEnable]
  Memory110/1 -> [Structure_M3_EtherCAT_PDO_ControlWord]
  Memory114/1 -> [Structure_M4_EtherCAT_SDO_6060_ModelEnable]
  Memory112/1 -> [Structure_M4_EtherCAT_SDO_6075_ModelEnable]
  Memory115/1 -> [Structure_M4_EtherCAT_SetDeviceState1_ModelEnable]
  Memory116/1 -> [Structure_M4_EtherCAT_GetDeviceState_ModelEnable]
  Memory117/1 -> [Structure_M4_EtherCAT_PDO_6040_ModelEnable]
  Memory118/1 -> [Structure_M4_EtherCAT_InitReadPos_ModelEnable]
  Memory119/1 -> [Structure_M4_EtherCAT_SetDeviceState_NewState]
  Memory120/1 -> [Structure_M4_EtherCAT_SetDeviceState_Enable]
  Memory124/1 -> [Structure_M4_EtherCAT_SDO_6060_Data]
  Memory123/1 -> [Structure_M4_EtherCAT_SDO_6080_Enable]
  Memory122/1 -> [Structure_M4_EtherCAT_SDO_6080_Data]
  Memory121/1 -> [Structure_M4_EtherCAT_SDO_6075_Enable]
  Memory126/1 -> [Structure_M4_EtherCAT_SetDeviceState1_NewState]
  Memory125/1 -> [Structure_M4_EtherCAT_SDO_6060_Enable]
  Memory127/1 -> [Structure_M4_EtherCAT_SetDeviceState1_Enable]
  Memory128/1 -> [Structure_M4_EtherCAT_PDO_ControlWord]
  Memory129/1 -> [Structure_EtherCAT_SlavePDORW_ModelEnable]
  Model/75 -> [Structure_M2_EtherCAT_PDO_DesireTorque]
  Model/76 -> [Structure_M3_EtherCAT_PDO_DesireTorque]
  Model/77 -> [Structure_M4_EtherCAT_PDO_DesireTorque]
  Model/78 -> [Structure_H_EtherCAT_PDO_Command]
  Model/74 -> [Structure_M1_EtherCAT_PDO_DesireTorque]
  Model/80 -> [Structure_H_EtherCAT_PDO_Data2]
  Model/79 -> [Structure_H_EtherCAT_PDO_Data1]
  Model/81 -> [Structure_H_EtherCAT_PDO_Data3]
  [Structure_M1_EtherCAT_PDO_VelocityActualValue] -> Model/59
  [Structure_M1_EtherCAT_PDO_TorqueActualValue] -> Model/60
  [Structure_M1_EtherCAT_PDO_PositionActualValue] -> Model/58
  [Structure_M1_EtherCAT_PDO_DCLinkCircuitVoltage] -> Model/61
  [Structure_M1_EtherCAT_PDO_ModeofOperationDisplay] -> Model/62
  [Structure_M2_EtherCAT_PDO_PositionActualValue] -> Model/63
  [Structure_M2_EtherCAT_PDO_VelocityActualValue] -> Model/64
  [Structure_M3_EtherCAT_PDO_TorqueActualValue] -> Model/70
  [Structure_M2_EtherCAT_PDO_TorqueActualValue] -> Model/65
  [Structure_M2_EtherCAT_PDO_DCLinkCircuitVoltage] -> Model/66
  [Structure_M3_EtherCAT_PDO_DCLinkCircuitVoltage] -> Model/71
  [Structure_M2_EtherCAT_PDO_ModeofOperationDisplay] -> Model/67
  [Structure_M3_EtherCAT_PDO_PositionActualValue] -> Model/68
  [Structure_M3_EtherCAT_PDO_VelocityActualValue] -> Model/69
  [Structure_M4_EtherCAT_PDO_PositionActualValue] -> Model/73
  [Structure_M3_EtherCAT_PDO_ModeofOperationDisplay] -> Model/72
  [Structure_M4_EtherCAT_PDO_ModeofOperationDisplay] -> Model/77
  [Structure_M4_EtherCAT_PDO_VelocityActualValue] -> Model/74
  [Structure_M4_EtherCAT_PDO_DCLinkCircuitVoltage] -> Model/76
  [Structure_M4_EtherCAT_PDO_TorqueActualValue] -> Model/75
  [Structure_S1_EtherCAT_PDO_ADch1] -> Model/78
  [Structure_S1_EtherCAT_PDO_q0] -> Model/80
  [Structure_S1_EtherCAT_PDO_ADch2] -> Model/79
  [Structure_S1_EtherCAT_PDO_q1] -> Model/81
  [Structure_S1_EtherCAT_PDO_q2] -> Model/82
  [Structure_S1_EtherCAT_PDO_q3] -> Model/83
  [Structure_S2_EtherCAT_PDO_ADch1] -> Model/84
  [Structure_S2_EtherCAT_PDO_ADch2] -> Model/85
  [Structure_S2_EtherCAT_PDO_q0] -> Model/86
  [Structure_S2_EtherCAT_PDO_q1] -> Model/87
  [Structure_S2_EtherCAT_PDO_q2] -> Model/88
  [Structure_S3_EtherCAT_PDO_ADch1] -> Model/90
  [Structure_S2_EtherCAT_PDO_q3] -> Model/89
  [Structure_S3_EtherCAT_PDO_q0] -> Model/92
  [Structure_S3_EtherCAT_PDO_ADch2] -> Model/91
  [Structure_S3_EtherCAT_PDO_q1] -> Model/93
  [Structure_S3_EtherCAT_PDO_q2] -> Model/94
  [Structure_S4_EtherCAT_PDO_ADch2] -> Model/97
  [Structure_S4_EtherCAT_PDO_q0] -> Model/98
  [Structure_S4_EtherCAT_PDO_ADch1] -> Model/96
  [Structure_S4_EtherCAT_PDO_q1] -> Model/99
  [Structure_S3_EtherCAT_PDO_q3] -> Model/95
  [Structure_S5_EtherCAT_PDO_ADch1] -> Model/102
  [Structure_S4_EtherCAT_PDO_q2] -> Model/100
  [Structure_S4_EtherCAT_PDO_q3] -> Model/101
  [Structure_S5_EtherCAT_PDO_ADch2] -> Model/103
  [Structure_S5_EtherCAT_PDO_q0] -> Model/104
  [Structure_S5_EtherCAT_PDO_q2] -> Model/106
  [Structure_S5_EtherCAT_PDO_q1] -> Model/105
  [Structure_S6_EtherCAT_PDO_ADch1] -> Model/108
  [Structure_S6_EtherCAT_PDO_q0] -> Model/110
  [Structure_S6_EtherCAT_PDO_q1] -> Model/111
  [Structure_S6_EtherCAT_PDO_q2] -> Model/112
  [Structure_S5_EtherCAT_PDO_q3] -> Model/107
  [Structure_S6_EtherCAT_PDO_ADch2] -> Model/109
  [Structure_S7_EtherCAT_PDO_ADch1] -> Model/114
  [Structure_S7_EtherCAT_PDO_q1] -> Model/117
  [Structure_S7_EtherCAT_PDO_q0] -> Model/116
  [Structure_S7_EtherCAT_PDO_ADch2] -> Model/115
  [Structure_S7_EtherCAT_PDO_q3] -> Model/119
  [Structure_S7_EtherCAT_PDO_q2] -> Model/118
  [Structure_H_EtherCAT_PDO_B1] -> Model/120
  [Structure_H_EtherCAT_PDO_B3] -> Model/122
  [Structure_H_EtherCAT_PDO_B5] -> Model/124
  [Structure_H_EtherCAT_PDO_B4] -> Model/123
  [Structure_H_EtherCAT_PDO_B2] -> Model/121
  [Structure_H_EtherCAT_PDO_B8] -> Model/125
  [Structure_H_EtherCAT_PDO_K1] -> Model/126
  [Structure_H_EtherCAT_PDO_K2] -> Model/127
  Model/83 -> BusIn/1
  [Structure_S6_EtherCAT_PDO_q3] -> Model/113
  Model/82 -> TaskEnable/1
  BusOut/1 -> Memory/1
  Memory/1 -> Model/129
  [Structure_H_EtherCAT_PDO_K3] -> Model/128
  MotorPositonInit1/2(i_d) -> Memory130/1
  MotorPositonInit1/1(TaskFinished) -> Memory131/1
  Model/84 -> MotorPositonInit1/Enable
  Model/85 -> MotorPositonInit1/1(P)
  Model/86 -> MotorPositonInit1/2(BusOut)
  Memory130/1 -> Model/131
  Memory131/1 -> Model/130
  [Structure_sEMG2_EtherCAT_PDO_ch1] -> Gain8/1
  [Structure_sEMG2_EtherCAT_PDO_ch0] -> Gain7/1
  [Structure_sEMG1_EtherCAT_PDO_ch2] -> Gain4/1
  [Structure_sEMG1_EtherCAT_PDO_ch3] -> Gain6/1
  [Structure_sEMG1_EtherCAT_PDO_ch0] -> Gain1/1
  [Structure_sEMG1_EtherCAT_PDO_ch1] -> Gain3/1
  Mux/1 -> sEMGMuxIn/1
  [Structure_sEMG2_EtherCAT_PDO_ch2] -> Gain5/1
  [Structure_sEMG2_EtherCAT_PDO_ch3] -> Gain9/1
  Gain1/1 -> Mux/1
  Gain3/1 -> Mux/2
  Gain4/1 -> Mux/3
  Gain5/1 -> Mux/7
  Gain6/1 -> Mux/4
  Gain7/1 -> Mux/5
  Gain8/1 -> Mux/6
  Gain9/1 -> Mux/8

== system TestStructure/Bus/Subsystem ==
  Enabled Subsystem : Subsystem  TreatAsAtomicUnit=on
  Enabled Subsystem1 : Subsystem  TreatAsAtomicUnit=on
  Enabled Subsystem2 : Subsystem  TreatAsAtomicUnit=on
  Enabled Subsystem3 : Subsystem  TreatAsAtomicUnit=on
  Enabled Subsystem4 : Subsystem  TreatAsAtomicUnit=on
  Enabled Subsystem5 : Subsystem  TreatAsAtomicUnit=on
  Enabled Subsystem6 : Subsystem  TreatAsAtomicUnit=on
  Enabled Subsystem7 : Subsystem  TreatAsAtomicUnit=on
  tag scope: Structure_M1_EtherCAT_GetDeviceState_State=global, Structure_M1_EtherCAT_Init_PDO_PositionActualValue=global, Structure_M1_EtherCAT_PDO_StatusWord=global, Structure_M1_EtherCAT_SDO_6060_Error=global, Structure_M1_EtherCAT_SDO_6060_Status=global, Structure_M1_EtherCAT_SDO_6075_Data=global, Structure_M1_EtherCAT_SDO_6075_Error=global, Structure_M1_EtherCAT_SDO_6075_Status=global, Structure_M1_EtherCAT_SDO_6080_Error=global, Structure_M1_EtherCAT_SDO_6080_Status=global, Structure_M1_EtherCAT_SetDeviceState1_Error=global, Structure_M1_EtherCAT_SetDeviceState1_PrevState=global, Structure_M1_EtherCAT_SetDeviceState_Error=global, Structure_M1_EtherCAT_SetDeviceState_PrevState=global
  wires:
  [Structure_M1_EtherCAT_SetDeviceState_ModelEnable] -> Enabled Subsystem/Enable
  [Structure_M1_EtherCAT_SDO_6075_ModelEnable] -> Enabled Subsystem1/Enable
  [Structure_M1_EtherCAT_SDO_6080_ModelEnable] -> Enabled Subsystem2/Enable
  [Structure_M1_EtherCAT_SDO_6060_ModelEnable] -> Enabled Subsystem3/Enable
  [Structure_M1_EtherCAT_SetDeviceState1_ModelEnable] -> Enabled Subsystem4/Enable
  [Structure_M1_EtherCAT_InitReadPos_ModelEnable] -> Enabled Subsystem7/Enable
  [Structure_M1_EtherCAT_PDO_6040_ModelEnable] -> Enabled Subsystem6/Enable
  [Structure_M1_EtherCAT_GetDeviceState_ModelEnable] -> Enabled Subsystem5/Enable
  [Structure_M1_EtherCAT_SetDeviceState_NewState] -> Enabled Subsystem/1(In1)
  [Structure_M1_EtherCAT_SetDeviceState_Enable] -> Enabled Subsystem/2(In2)
  Enabled Subsystem/1(Out1) -> [Structure_M1_EtherCAT_SetDeviceState_PrevState]
  Enabled Subsystem/2(Out2) -> [Structure_M1_EtherCAT_SetDeviceState_Error]
  [Structure_M1_EtherCAT_SDO_6075_Enable] -> Enabled Subsystem1/1(In3)
  Enabled Subsystem1/1(Out3) -> [Structure_M1_EtherCAT_SDO_6075_Data]
  Enabled Subsystem1/2(Out4) -> [Structure_M1_EtherCAT_SDO_6075_Status]
  Enabled Subsystem1/3(Out5) -> [Structure_M1_EtherCAT_SDO_6075_Error]
  [Structure_M1_EtherCAT_SDO_6080_Enable] -> Enabled Subsystem2/2(In5)
  [Structure_M1_EtherCAT_SDO_6080_Data] -> Enabled Subsystem2/1(In4)
  Enabled Subsystem2/2(Out7) -> [Structure_M1_EtherCAT_SDO_6080_Error]
  Enabled Subsystem2/1(Out6) -> [Structure_M1_EtherCAT_SDO_6080_Status]
  [Structure_M1_EtherCAT_SDO_6060_Data] -> Enabled Subsystem3/1(In6)
  [Structure_M1_EtherCAT_SDO_6060_Enable] -> Enabled Subsystem3/2(In7)
  Enabled Subsystem3/1(Out8) -> [Structure_M1_EtherCAT_SDO_6060_Status]
  Enabled Subsystem3/2(Out9) -> [Structure_M1_EtherCAT_SDO_6060_Error]
  [Structure_M1_EtherCAT_SetDeviceState1_NewState] -> Enabled Subsystem4/1(In8)
  [Structure_M1_EtherCAT_SetDeviceState1_Enable] -> Enabled Subsystem4/2(In9)
  Enabled Subsystem4/1(Out10) -> [Structure_M1_EtherCAT_SetDeviceState1_PrevState]
  Enabled Subsystem4/2(Out11) -> [Structure_M1_EtherCAT_SetDeviceState1_Error]
  Enabled Subsystem5/1(Out12) -> [Structure_M1_EtherCAT_GetDeviceState_State]
  [Structure_M1_EtherCAT_PDO_ControlWord] -> Enabled Subsystem6/1(In10)
  Enabled Subsystem6/1(Out13) -> [Structure_M1_EtherCAT_PDO_StatusWord]
  Enabled Subsystem7/1(Out1) -> [Structure_M1_EtherCAT_Init_PDO_PositionActualValue]

== system TestStructure/Bus/Subsystem1 ==
  "DCErrVal " : Display
  "DCInitState " : Display
  Demux : Demux  Outputs=6
  "ErrVal " : Display
  EtherCAT Init : slrealtimeethercatlib/EtherCAT Init  Priority=0  config_file=C:\Users\My-Dell-PC\OneDrive\PC\Pro-HemiplegiaRehabilitationExoskeleton\Code\TestStructure10-release-zhuyu-Revise03\HemiplegiaRehabilitationExoskeleton_ESI.xml  device_id=0  portnum=1  initstate=2  dctuning=0  enaDebug=1  logFile='c:\dbglog.txt'  sample_time=0.001000  DCMode=1
  "MasterState " : Display
  "MasterToNetworkClkDiff " : Display
  "NetworkToSlaveClkDiff " : Display
  tag scope: Structure_EtherCAT_Init=global
  wires:
  Demux/4 -> "MasterToNetworkClkDiff "/1
  Demux/1 -> "ErrVal "/1
  Demux/5 -> "DCInitState "/1
  Demux/3 -> "DCErrVal "/1
  EtherCAT Init/1 -> Demux/1, [Structure_EtherCAT_Init]
  Demux/2 -> "MasterState "/1
  Demux/6 -> "NetworkToSlaveClkDiff "/1

== system TestStructure/Bus/Subsystem4 ==
  Enabled Subsystem : Subsystem  TreatAsAtomicUnit=on
  Enabled Subsystem1 : Subsystem  TreatAsAtomicUnit=on
  Enabled Subsystem2 : Subsystem  TreatAsAtomicUnit=on
  Enabled Subsystem3 : Subsystem  TreatAsAtomicUnit=on
  Enabled Subsystem4 : Subsystem  TreatAsAtomicUnit=on
  Enabled Subsystem5 : Subsystem  TreatAsAtomicUnit=on
  Enabled Subsystem6 : Subsystem  TreatAsAtomicUnit=on
  Enabled Subsystem7 : Subsystem  TreatAsAtomicUnit=on
  tag scope: Structure_M2_EtherCAT_GetDeviceState_State=global, Structure_M2_EtherCAT_Init_PDO_PositionActualValue=global, Structure_M2_EtherCAT_PDO_StatusWord=global, Structure_M2_EtherCAT_SDO_6060_Error=global, Structure_M2_EtherCAT_SDO_6060_Status=global, Structure_M2_EtherCAT_SDO_6075_Data=global, Structure_M2_EtherCAT_SDO_6075_Error=global, Structure_M2_EtherCAT_SDO_6075_Status=global, Structure_M2_EtherCAT_SDO_6080_Error=global, Structure_M2_EtherCAT_SDO_6080_Status=global, Structure_M2_EtherCAT_SetDeviceState1_Error=global, Structure_M2_EtherCAT_SetDeviceState1_PrevState=global, Structure_M2_EtherCAT_SetDeviceState_Error=global, Structure_M2_EtherCAT_SetDeviceState_PrevState=global
  wires:
  [Structure_M2_EtherCAT_SetDeviceState_ModelEnable] -> Enabled Subsystem/Enable
  [Structure_M2_EtherCAT_SDO_6075_ModelEnable] -> Enabled Subsystem1/Enable
  [Structure_M2_EtherCAT_SDO_6080_ModelEnable] -> Enabled Subsystem2/Enable
  [Structure_M2_EtherCAT_SDO_6060_ModelEnable] -> Enabled Subsystem3/Enable
  [Structure_M2_EtherCAT_SetDeviceState1_ModelEnable] -> Enabled Subsystem4/Enable
  [Structure_M2_EtherCAT_InitReadPos_ModelEnable] -> Enabled Subsystem7/Enable
  [Structure_M2_EtherCAT_PDO_6040_ModelEnable] -> Enabled Subsystem6/Enable
  [Structure_M2_EtherCAT_GetDeviceState_ModelEnable] -> Enabled Subsystem5/Enable
  [Structure_M2_EtherCAT_SetDeviceState_NewState] -> Enabled Subsystem/1(In1)
  [Structure_M2_EtherCAT_SetDeviceState_Enable] -> Enabled Subsystem/2(In2)
  Enabled Subsystem/1(Out1) -> [Structure_M2_EtherCAT_SetDeviceState_PrevState]
  Enabled Subsystem/2(Out2) -> [Structure_M2_EtherCAT_SetDeviceState_Error]
  [Structure_M2_EtherCAT_SDO_6075_Enable] -> Enabled Subsystem1/1(In3)
  Enabled Subsystem1/1(Out3) -> [Structure_M2_EtherCAT_SDO_6075_Data]
  Enabled Subsystem1/2(Out4) -> [Structure_M2_EtherCAT_SDO_6075_Status]
  Enabled Subsystem1/3(Out5) -> [Structure_M2_EtherCAT_SDO_6075_Error]
  [Structure_M2_EtherCAT_SDO_6080_Enable] -> Enabled Subsystem2/2(In5)
  [Structure_M2_EtherCAT_SDO_6080_Data] -> Enabled Subsystem2/1(In4)
  Enabled Subsystem2/2(Out7) -> [Structure_M2_EtherCAT_SDO_6080_Error]
  Enabled Subsystem2/1(Out6) -> [Structure_M2_EtherCAT_SDO_6080_Status]
  [Structure_M2_EtherCAT_SDO_6060_Data] -> Enabled Subsystem3/1(In6)
  [Structure_M2_EtherCAT_SDO_6060_Enable] -> Enabled Subsystem3/2(In7)
  Enabled Subsystem3/1(Out8) -> [Structure_M2_EtherCAT_SDO_6060_Status]
  Enabled Subsystem3/2(Out9) -> [Structure_M2_EtherCAT_SDO_6060_Error]
  [Structure_M2_EtherCAT_SetDeviceState1_NewState] -> Enabled Subsystem4/1(In8)
  [Structure_M2_EtherCAT_SetDeviceState1_Enable] -> Enabled Subsystem4/2(In9)
  Enabled Subsystem4/1(Out10) -> [Structure_M2_EtherCAT_SetDeviceState1_PrevState]
  Enabled Subsystem4/2(Out11) -> [Structure_M2_EtherCAT_SetDeviceState1_Error]
  Enabled Subsystem5/1(Out12) -> [Structure_M2_EtherCAT_GetDeviceState_State]
  [Structure_M2_EtherCAT_PDO_ControlWord] -> Enabled Subsystem6/1(In10)
  Enabled Subsystem6/1(Out13) -> [Structure_M2_EtherCAT_PDO_StatusWord]
  Enabled Subsystem7/1(Out1) -> [Structure_M2_EtherCAT_Init_PDO_PositionActualValue]

== system TestStructure/Bus/Subsystem5 ==
  Enabled Subsystem : Subsystem  Commented=on  TreatAsAtomicUnit=on
  Enabled Subsystem1 : Subsystem  Commented=on  TreatAsAtomicUnit=on
  Enabled Subsystem2 : Subsystem  Commented=on  TreatAsAtomicUnit=on
  Enabled Subsystem3 : Subsystem  Commented=on  TreatAsAtomicUnit=on
  Enabled Subsystem4 : Subsystem  Commented=on  TreatAsAtomicUnit=on
  Enabled Subsystem5 : Subsystem  Commented=on  TreatAsAtomicUnit=on
  Enabled Subsystem6 : Subsystem  Commented=on  TreatAsAtomicUnit=on
  Enabled Subsystem7 : Subsystem  Commented=on  TreatAsAtomicUnit=on
  tag scope: Structure_M3_EtherCAT_GetDeviceState_State=global, Structure_M3_EtherCAT_Init_PDO_PositionActualValue=global, Structure_M3_EtherCAT_PDO_StatusWord=global, Structure_M3_EtherCAT_SDO_6060_Error=global, Structure_M3_EtherCAT_SDO_6060_Status=global, Structure_M3_EtherCAT_SDO_6075_Data=global, Structure_M3_EtherCAT_SDO_6075_Error=global, Structure_M3_EtherCAT_SDO_6075_Status=global, Structure_M3_EtherCAT_SDO_6080_Error=global, Structure_M3_EtherCAT_SDO_6080_Status=global, Structure_M3_EtherCAT_SetDeviceState1_Error=global, Structure_M3_EtherCAT_SetDeviceState1_PrevState=global, Structure_M3_EtherCAT_SetDeviceState_Error=global, Structure_M3_EtherCAT_SetDeviceState_PrevState=global
  wires:
  [Structure_M3_EtherCAT_SetDeviceState_ModelEnable] -> Enabled Subsystem/Enable
  [Structure_M3_EtherCAT_SDO_6075_ModelEnable] -> Enabled Subsystem1/Enable
  [Structure_M3_EtherCAT_SDO_6080_ModelEnable] -> Enabled Subsystem2/Enable
  [Structure_M3_EtherCAT_SDO_6060_ModelEnable] -> Enabled Subsystem3/Enable
  [Structure_M3_EtherCAT_SetDeviceState1_ModelEnable] -> Enabled Subsystem4/Enable
  [Structure_M3_EtherCAT_InitReadPos_ModelEnable] -> Enabled Subsystem7/Enable
  [Structure_M3_EtherCAT_PDO_6040_ModelEnable] -> Enabled Subsystem6/Enable
  [Structure_M3_EtherCAT_GetDeviceState_ModelEnable] -> Enabled Subsystem5/Enable
  [Structure_M3_EtherCAT_SetDeviceState_NewState] -> Enabled Subsystem/1(In1)
  [Structure_M3_EtherCAT_SetDeviceState_Enable] -> Enabled Subsystem/2(In2)
  Enabled Subsystem/1(Out1) -> [Structure_M3_EtherCAT_SetDeviceState_PrevState]
  Enabled Subsystem/2(Out2) -> [Structure_M3_EtherCAT_SetDeviceState_Error]
  [Structure_M3_EtherCAT_SDO_6075_Enable] -> Enabled Subsystem1/1(In3)
  Enabled Subsystem1/1(Out3) -> [Structure_M3_EtherCAT_SDO_6075_Data]
  Enabled Subsystem1/2(Out4) -> [Structure_M3_EtherCAT_SDO_6075_Status]
  Enabled Subsystem1/3(Out5) -> [Structure_M3_EtherCAT_SDO_6075_Error]
  [Structure_M3_EtherCAT_SDO_6080_Enable] -> Enabled Subsystem2/2(In5)
  [Structure_M3_EtherCAT_SDO_6080_Data] -> Enabled Subsystem2/1(In4)
  Enabled Subsystem2/2(Out7) -> [Structure_M3_EtherCAT_SDO_6080_Error]
  Enabled Subsystem2/1(Out6) -> [Structure_M3_EtherCAT_SDO_6080_Status]
  [Structure_M3_EtherCAT_SDO_6060_Data] -> Enabled Subsystem3/1(In6)
  [Structure_M3_EtherCAT_SDO_6060_Enable] -> Enabled Subsystem3/2(In7)
  Enabled Subsystem3/1(Out8) -> [Structure_M3_EtherCAT_SDO_6060_Status]
  Enabled Subsystem3/2(Out9) -> [Structure_M3_EtherCAT_SDO_6060_Error]
  [Structure_M3_EtherCAT_SetDeviceState1_NewState] -> Enabled Subsystem4/1(In8)
  [Structure_M3_EtherCAT_SetDeviceState1_Enable] -> Enabled Subsystem4/2(In9)
  Enabled Subsystem4/1(Out10) -> [Structure_M3_EtherCAT_SetDeviceState1_PrevState]
  Enabled Subsystem4/2(Out11) -> [Structure_M3_EtherCAT_SetDeviceState1_Error]
  Enabled Subsystem5/1(Out12) -> [Structure_M3_EtherCAT_GetDeviceState_State]
  [Structure_M3_EtherCAT_PDO_ControlWord] -> Enabled Subsystem6/1(In10)
  Enabled Subsystem6/1(Out13) -> [Structure_M3_EtherCAT_PDO_StatusWord]
  Enabled Subsystem7/1(Out1) -> [Structure_M3_EtherCAT_Init_PDO_PositionActualValue]
